simulink library "dlbsBlockSplit"  (R2025b)
settings: Solver=VariableStepAuto  StartTime=0.0  StopTime=10.0  RelTol=1e-3
libraries: dlbsBlockExtractGradientGF x10, $bdroot x10, dlbsBlockInsertGradientGF x4
settings Model: Creator=lt6037  LastModifiedBy=lt6037

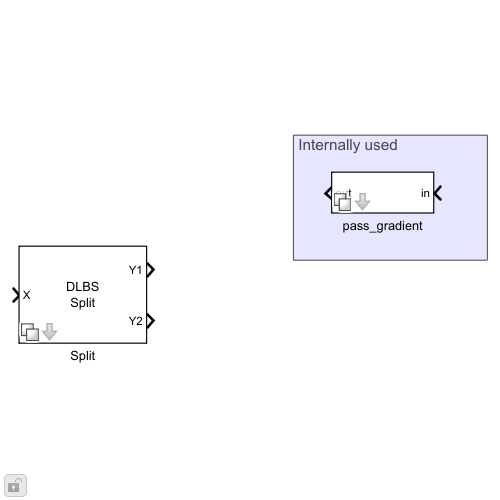
[thumbnail: Simulink's stored preview of the top-level diagram]
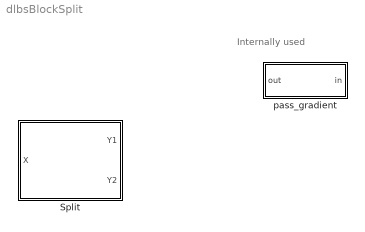
== system dlbsBlockSplit ==
  note: Internally used
  Split : Subsystem  Variant=on  mask{n_out=2, g1=on, g2=on, g3=on, g4=on}
      mask prompts: n_out "Number of outputs"; g1 "Output 1"; g2 "Output 2"; g3 "Output 3"; g4 "Output 4"
      mask help: Copies one input tensor to multiple outputs. The input gradient is computed as the sum of contributing output gradients.
      mask Help: web("dlbsHelpBlockSplit.html")
      mask TypeOptions g1: n1/g1 | n2/g1 | n3/g1 | n4/g1
      mask TypeOptions g2: n2/g2 | n3/g2 | n4/g2
      mask TypeOptions g3: n3/g3 | n4/g3
      mask TypeOptions g4: n4/g4
      mask DialogControl Container3 Prompt: Outputs contributing to the gradient of the index
      mask Display: disp("DLBS\nSplit")
  pass_gradient : Subsystem  Variant=on  mask{pass_gradient=on}
      mask prompts: pass_gradient "Pass gradient"

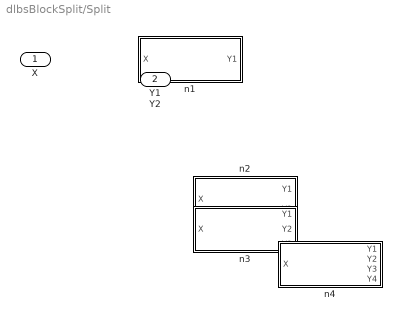
== system dlbsBlockSplit/Split ==
  X : Inport
  n1 : Subsystem  VariantControl=n_out==1  mask{g1=on}
      mask TypeOptions g1: g1/pass_gradient
  n2 : Subsystem  VariantControl=n_out==2  mask{g1=on, g2=on}
      mask TypeOptions g1: g1/pass_gradient
      mask TypeOptions g2: g2/pass_gradient
  n3 : Subsystem  VariantControl=n_out==3  mask{g1=on, g2=on, g3=on}
      mask TypeOptions g1: g1/pass_gradient
      mask TypeOptions g2: g2/pass_gradient
      mask TypeOptions g3: g3/pass_gradient
  n4 : Subsystem  VariantControl=n_out==4  mask{g1=on, g2=on, g3=on, g4=on}
      mask TypeOptions g1: g1/pass_gradient
      mask TypeOptions g2: g2/pass_gradient
      mask TypeOptions g3: g3/pass_gradient
      mask TypeOptions g4: g4/pass_gradient
  Y1 : Outport
  Y2 : Outport  Port=2

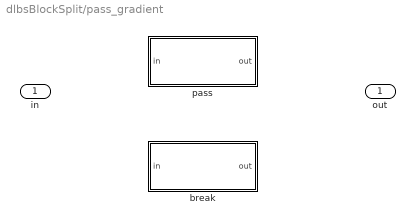
== system dlbsBlockSplit/pass_gradient ==
  in : Inport
  break : Subsystem  VariantControl=pass_gradient==false
  pass : Subsystem  VariantControl=pass_gradient==true
  out : Outport

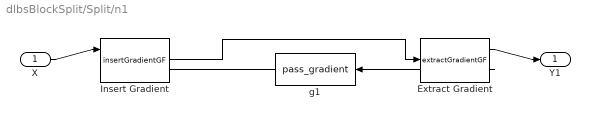
== system dlbsBlockSplit/Split/n1 ==
  X : Inport
  Extract Gradient : dlbsBlockExtractGradientGF/extractGradientGF
  Insert Gradient : dlbsBlockInsertGradientGF/insertGradientGF
  g1 : $bdroot/pass_gradient  pass_gradient=on
  Y1 : Outport
  wires:
  Insert Gradient/1 -> Extract Gradient/1
  Extract Gradient/2 -> g1/1
  g1/1 -> Insert Gradient/2
  X/1 -> Insert Gradient/1
  Extract Gradient/1 -> Y1/1

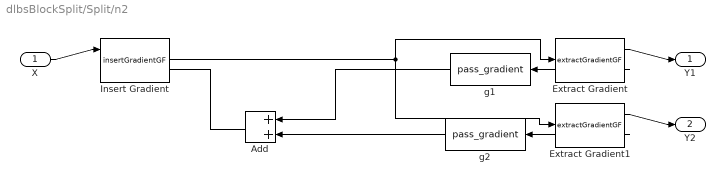
== system dlbsBlockSplit/Split/n2 ==
  X : Inport
  Add : Sum
  Extract Gradient : dlbsBlockExtractGradientGF/extractGradientGF
  Extract Gradient1 : dlbsBlockExtractGradientGF/extractGradientGF
  Insert Gradient : dlbsBlockInsertGradientGF/insertGradientGF
  g1 : $bdroot/pass_gradient  pass_gradient=on
  g2 : $bdroot/pass_gradient  pass_gradient=on
  Y1 : Outport
  Y2 : Outport  Port=2
  wires:
  Add/1 -> Insert Gradient/2
  Insert Gradient/1 -> Extract Gradient/1, Extract Gradient1/1
  Extract Gradient1/2 -> g2/1
  Extract Gradient/2 -> g1/1
  g1/1 -> Add/1
  g2/1 -> Add/2
  X/1 -> Insert Gradient/1
  Extract Gradient/1 -> Y1/1
  Extract Gradient1/1 -> Y2/1

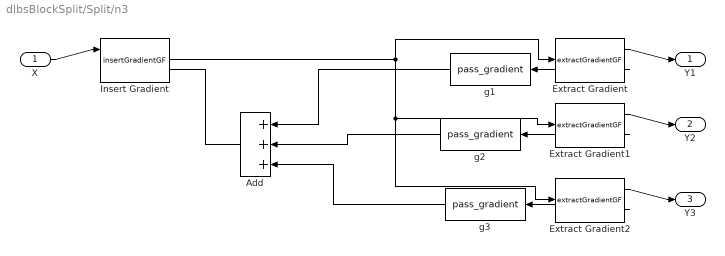
== system dlbsBlockSplit/Split/n3 ==
  X : Inport
  Add : Sum  Inputs=+++
  Extract Gradient : dlbsBlockExtractGradientGF/extractGradientGF
  Extract Gradient1 : dlbsBlockExtractGradientGF/extractGradientGF
  Extract Gradient2 : dlbsBlockExtractGradientGF/extractGradientGF
  Insert Gradient : dlbsBlockInsertGradientGF/insertGradientGF
  g1 : $bdroot/pass_gradient  pass_gradient=on
  g2 : $bdroot/pass_gradient  pass_gradient=on
  g3 : $bdroot/pass_gradient  pass_gradient=on
  Y1 : Outport
  Y2 : Outport  Port=2
  Y3 : Outport  Port=3
  wires:
  Add/1 -> Insert Gradient/2
  Insert Gradient/1 -> Extract Gradient/1, Extract Gradient2/1, Extract Gradient1/1
  Extract Gradient1/2 -> g2/1
  Extract Gradient/2 -> g1/1
  g1/1 -> Add/1
  g2/1 -> Add/2
  Extract Gradient2/2 -> g3/1
  g3/1 -> Add/3
  X/1 -> Insert Gradient/1
  Extract Gradient/1 -> Y1/1
  Extract Gradient1/1 -> Y2/1
  Extract Gradient2/1 -> Y3/1

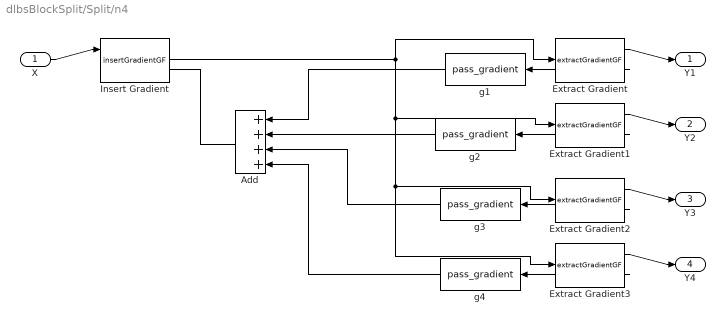
== system dlbsBlockSplit/Split/n4 ==
  X : Inport
  Add : Sum  Inputs=++++
  Extract Gradient{,1..3} (4 alike) : dlbsBlockExtractGradientGF/extractGradientGF
  Insert Gradient : dlbsBlockInsertGradientGF/insertGradientGF
  g{1..4} (4 alike) : $bdroot/pass_gradient  pass_gradient=on
  Y1 : Outport
  Y2 : Outport  Port=2
  Y3 : Outport  Port=3
  Y4 : Outport  Port=4
  wires:
  Add/1 -> Insert Gradient/2
  Insert Gradient/1 -> Extract Gradient/1, Extract Gradient3/1, Extract Gradient2/1, Extract Gradient1/1
  Extract Gradient1/2 -> g2/1
  Extract Gradient/2 -> g1/1
  g1/1 -> Add/1
  g2/1 -> Add/2
  Extract Gradient2/2 -> g3/1
  Extract Gradient3/2 -> g4/1
  g3/1 -> Add/3
  g4/1 -> Add/4
  X/1 -> Insert Gradient/1
  Extract Gradient3/1 -> Y4/1
  Extract Gradient2/1 -> Y3/1
  Extract Gradient1/1 -> Y2/1
  Extract Gradient/1 -> Y1/1

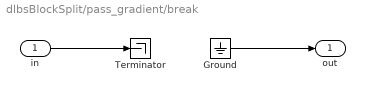
== system dlbsBlockSplit/pass_gradient/break ==
  in : Inport
  Ground : Ground
  Terminator : Terminator
  out : Outport
  wires:
  in/1 -> Terminator/1
  Ground/1 -> out/1

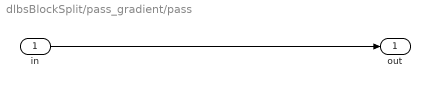
== system dlbsBlockSplit/pass_gradient/pass ==
  in : Inport
  out : Outport
  wires:
  in/1 -> out/1
